simulink model "ap"  (R2025b)
settings: Solver=FixedStepDiscrete  StartTime=0.0  StopTime=10.0  RelTol=1e-3
settings Model: Creator=matthewkeller  LastModifiedBy=ryanj
settings OptimizationCC: DefaultParameterBehavior=Inlined  EnhancedBackFolding=on  PassReuseOutputArgsThreshold=0.0  ZeroExternalMemoryAtStartup=off  ZeroInternalMemoryAtStartup=off  OptimizeBlockOrder=speed  DifferentSizesBufferReuse=on  OptimizationCustomize=off
settings DebuggingCC: ParameterTunabilityLossMsg=error
settings SFSimCC: MATLABDynamicMemAlloc=off
settings RTWCC: SystemTargetFile=rtmaps.tlc  TemplateMakefile=rtmaps_default_tmf  RetainRTWFile=on  TargetLang=C++  Description=Generate an RTMaps component embedding the model
settings CodeAppCC: ForceParamTrailComments=on  OperatorAnnotations=on
settings STFCustomTargetCC: SystemTargetFile=rtmaps.tlc  TargetLangStandard=C++11 (ISO)  ModelReferenceCompliant=off  CombineOutputUpdateFcns=on  CodeInterfacePackaging=C++ class  SubcomponentCodeInterfacePackaging=C++ class  CPPClassGenCompliant=on  GRTInterface=off  RTMaps_GRTInterface=0  RTMaps_MultiInstanceCode=1  RTMAPS_BOARD=vc.net2022_x64  RTMaps_CombineOutputUpdateFcns=1  RTMAPS_OS=vc.net2022  RTMAPS_ARCH=x86_64  DisplayOptimOptions=off  RTMAPS_SDKDIR=C:\Program Files\Intempora\RTMaps 4  CustomFileTemplate=rtmaps_file_process.tlc  RTMaps_GenerateAllocFcn=0  RTMaps_MatFileLogging=0  RTMaps_GenerateERTSFunction=0  RTMaps_IntegerCode=0
settings GRTTargetCC: TargetLangStandard=C++11 (ISO)  ModelReferenceCompliant=off  ParMdlRefBuildCompliant=off  CompOptLevelCompliant=off  MatFileLogging=off  CodeInterfacePackaging=C++ class  SubcomponentCodeInterfacePackaging=C++ class  UseToolchainInfoCompliant=off

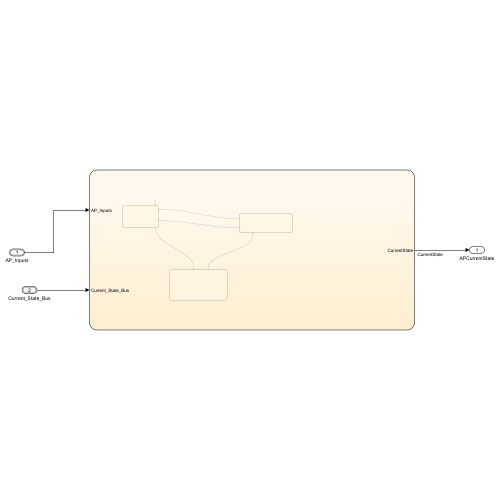
[thumbnail: Simulink's stored preview of the top-level diagram]
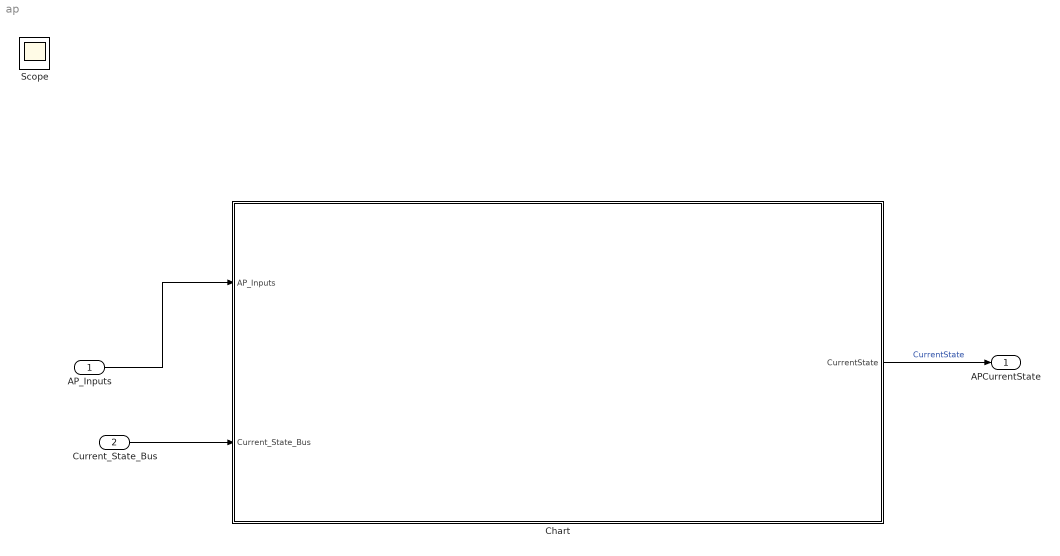
== system ap ==
  AP_Inputs : Inport  OutDataTypeStr=Bus: APStatusBus
  Current_State_Bus : Inport  Port=2  OutDataTypeStr=Bus: CurrentStateBus
  Chart : Stateflow chart  TreatAsAtomicUnit=on
  APCurrentState : Outport
  Scope : Scope
      settings: ActiveDisplayYMinimum=-1  ActiveDisplayYMaximum=1
  wires:
  Chart/1(CurrentState) -> APCurrentState/1  "CurrentState"
  AP_Inputs/1 -> Chart/1(AP_Inputs)
  Current_State_Bus/1 -> Chart/2(Current_State_Bus)

== stateflow chart ap/Chart ==
  settings: executeAtInitialization=1
  state AP_Deactivated
    entry:
    CurrentState = StatusType.Deactivated;
  state AP_Active
    entry:
    CurrentState = StatusType.Active;
  state AP_Standby
    entry:
    CurrentState = StatusType.Standby;
  (default) -> AP_Deactivated
  AP_Active -> AP_Deactivated [order 1] : [AP_Inputs.Cancel_AP_Pressed]
  AP_Active -> AP_Deactivated [order 2] : [AP_Inputs.Finish_Pressed]
  AP_Deactivated -> AP_Standby : [AP_Inputs.Longitudinal_Switch_ON && AP_Inputs.Lateral_Switch_ON && AP_Inputs.Driver_Brakes && AP_Inputs.Is_Stationary && Current_State_Bus.AINStatus == 0 && Current_State_Bus.ACCStatus == 0 && Current_State_Bus.CACCStatus == 0 && Current_State_Bus.LCCStatus == 0]
  AP_Standby -> AP_Active : [AP_Inputs.Activate_AP_Pressed && AP_Inputs.Parking_In_Range]
  data: CurrentState output Enum: StatusType; AP_Inputs input; Current_State_Bus input Bus: CurrentStateBus
